simulink model "BetaCal"  (R2022b)
settings: Solver=VariableStepAuto  StartTime=0.0  StopTime=1000  RelTol=1e-3
settings Model: Creator=Lenovo  LastModifiedBy=Lenovo

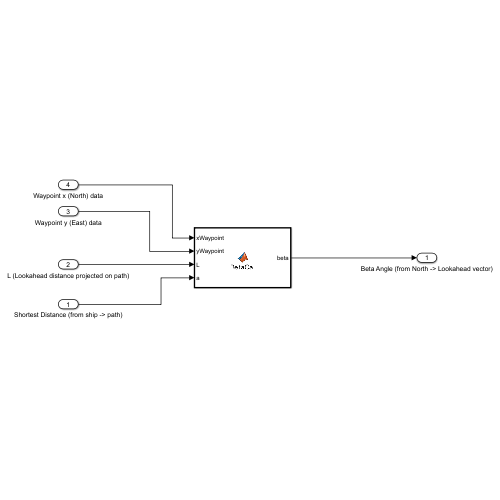
[thumbnail: Simulink's stored preview of the top-level diagram]
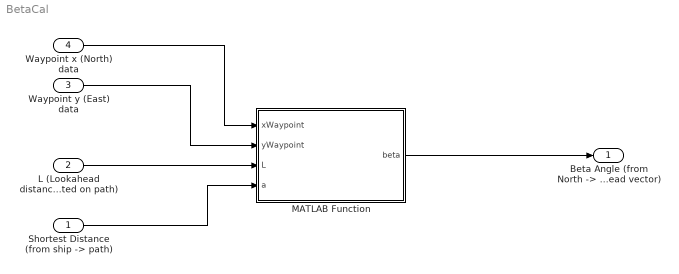
== system BetaCal ==
  "Shortest Distance (from ship -> path)" : Inport
  L (Lookahead distance projected on path) : Inport  Port=2
  Waypoint y (East) data : Inport  Port=3
  Waypoint x (North) data : Inport  Port=4
  MATLAB Function : MATLAB Function  TreatAsAtomicUnit=on
  "Beta Angle (from North -> Lookahead vector)" : Outport
  wires:
  MATLAB Function/1(beta) -> "Beta Angle (from North -> Lookahead vector)"/1
  Waypoint x (North) data/1 -> MATLAB Function/1(xWaypoint)
  Waypoint y (East) data/1 -> MATLAB Function/2(yWaypoint)
  L (Lookahead distance projected on path)/1 -> MATLAB Function/3(L)
  "Shortest Distance (from ship -> path)"/1 -> MATLAB Function/4(a)

== matlab function BetaCal/MATLAB Function ==
  data: xWaypoint input; yWaypoint input; beta output; L input; a input
function beta = BetaCal(xWaypoint,yWaypoint,L,a)

% line coefficient
alpha = atan2((xWaypoint(2) - xWaypoint(1)) / (yWaypoint(2) - yWaypoint(1)));

beta = atan2(L/a) - alpha;
